simulink model "CAN_Tx"  (R2019b)
settings: Solver=FixedStepDiscrete  StartTime=0.0  StopTime=Inf  RelTol=1e-3  EnableMultiTasking=on
libraries: c2837xDlib x2, drivingvehiclecontroller x1, canmsglib x1, c280xlib x1
settings Model: ExtModeTrigDuration=8  Creator=The MathWorks, Inc.  LastModifiedBy=hang
settings DataIOCC: LimitDataPoints=on  SaveFormat=Array  SaveOutput=off  SaveTime=off  ReturnWorkspaceOutputs=off
settings OptimizationCC: DefaultUnderspecifiedDataType=single  ExpressionDepthLimit=2147483647  LifeSpan=1  MaxStackSize=1024  DenormalBehavior=FlushToZero  EfficientTunableParamExpr=on
settings DebuggingCC: UnderspecifiedInitializationDetection=Classic  MergeDetectMultiDrivingBlocksExec=none  SolverPrmCheckMsg=warning  FcnCallInpInsideContextMsg=warning  AllowSymbolicDim=off  StateNameClashWarn=warning  SFUnexpectedBacktrackingDiag=warning  SFNoUnconditionalDefaultTransitionDiag=warning  SFExecutionAtInitializationDiag=none  ArithmeticOperatorsInVariantConditions=warning
settings HardwareCC: ProdBitPerChar=16  ProdBitPerInt=16  ProdBitPerPointer=32  ProdBitPerSizeT=32  ProdBitPerPtrDiffT=32  ProdLargestAtomicInteger=Integer  ProdLargestAtomicFloat=None  ProdWordSize=16  ProdLongLongMode=on  ProdHWDeviceType=Texas Instruments->C2000
settings ModelReferenceCC: PropagateSignalLabelsOutOfModel=off
settings SFSimCC: SimUseLocalCustomCode=off  MATLABDynamicMemAlloc=off  CustomCodeUndefinedFunction=UseInterfaceOnly
settings RTWCC: SystemTargetFile=ert.tlc  HardwareBoard=TI Delfino F28379D LaunchPad  TemplateMakefile=ert_default_tmf  RTWUseLocalCustomCode=off  Toolchain=Texas Instruments Code Composer Studio (C2000)
settings CodeAppCC: IgnoreCustomStorageClasses=off  CustomSymbolStrType=$N$R$M  StateflowObjectComments=on  InternalIdentifier=Classic
settings ERTTargetCC: CodeReplacementLibrary=TI C28x  MultiwordLength=2048  ExtModeStaticAllocSize=10000  ConvertIfToSwitch=off  SuppressUnreachableDefaultCases=off
settings ConfigComp: CovMetricSettings=dw  CovHtmlReporting=on  CovSaveCumulativeToWorkspaceVar=on  CovSaveSingleToWorkspaceVar=on  CovExternalEMLEnable=off

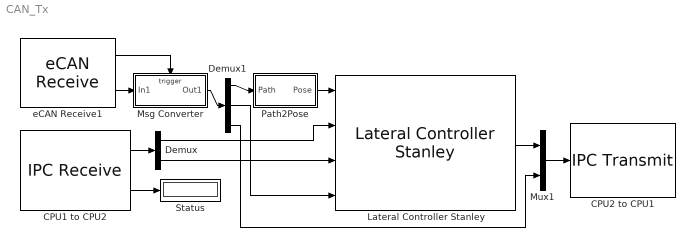
== system CAN_Tx ==
  CPU1 to CPU2 : c2837xDlib/IPC Receive  SelectChannel=1  DataType=uint32  DataLength=1  EnableBlocking=off  SampleTime=0.2
      settings: SourceProductName=Embedded Coder Support Package for Texas Instruments C2000 Processors  SourceProductBaseCode=TIC2000
  CPU2 to CPU1 : c2837xDlib/IPC Transmit  SelectChannel=0  EnableBlocking=off
      settings: SourceProductName=Embedded Coder Support Package for Texas Instruments C2000 Processors  SourceProductBaseCode=TIC2000
  Demux : Demux  Outputs=2
  Demux1 : Demux  Outputs=3
  Lateral Controller Stanley : drivingvehiclecontroller/Lateral Controller Stanley  ModelType=Kinematic bicycle model  PositionGainF=2.5  PositionGainR=2.5  YawRateGain=0.2  DelayGain=0.2  VehicleMass=1575  Lf=1.2  Lr=1.6  TireStiffness=19000  Wheelbase=2.8  MaxSteeringAngle=35
      settings: SourceProductName=Automated Driving Toolbox  SourceProductBaseCode=DR
  Msg Converter : Subsystem  TreatAsAtomicUnit=on
  Mux1 : Mux  Inputs=2
  Path2Pose : Subsystem
  Status : Display
  eCAN Receive1 : c280xlib/eCAN Receive  chipFamily=C280x  useModule=eCAN_B  mailboxNo=0  messageID=bin2dec('1')  messageType=Standard (11-bit identifier)  sampleTime=0.005  dataType=CAN_MESSAGE_TYPE  initValue=0  outputMessageLength=off  outputMessageTimeStamp=off  postInterrupt=off  interruptLine=0
      settings: SourceProductName=Embedded Coder Support Package for Texas Instruments C2000 Processors  SourceProductBaseCode=TIC2000
  wires:
  eCAN Receive1/2 -> Msg Converter/1(In1)
  eCAN Receive1/1 -> Msg Converter/Trigger
  Path2Pose/1(Pose) -> Lateral Controller Stanley/1
  CPU1 to CPU2/1 -> Demux/1
  Demux/1 -> Lateral Controller Stanley/2
  Demux/2 -> Lateral Controller Stanley/3
  CPU1 to CPU2/2 -> Status/1
  Mux1/1 -> CPU2 to CPU1/1
  Lateral Controller Stanley/1 -> Mux1/1
  Demux1/1 -> Path2Pose/1(Path)
  Msg Converter/1(Out1) -> Demux1/1
  Demux1/2 -> Lateral Controller Stanley/4
  Demux1/3 -> Mux1/2

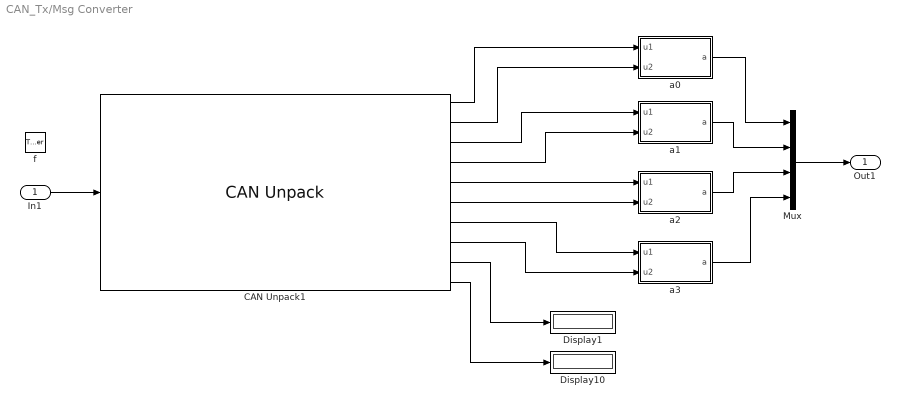
== system CAN_Tx/Msg Converter ==
  In1 : Inport
  f : TriggerPort  TriggerType=function-call  VariantControl=Variant
  CAN Unpack1 : canmsglib/CAN Unpack  MsgList=(none)  MsgName=CAN Msg  MsgIDType=Standard (11-bit identifier)  MsgIdentifier=bin2dec('1')  MsgLength=8  SignalInfo={ 'Signal1', '0', '8', 'LE', 'unsigned', 'Standard', '0', '1', '0', '0', '255'; 'Signal2', '8', '8', 'LE', 'unsigned', 'Standard', '0', '1', '0', '0', '255'; 'Signal3', '16', '8', 'LE', 'unsigned', 'Standard', '0', '1', '0', '0', '255'; 'Signal4', '24', '8', 'LE', 'unsigned', 'Standard', '0', '1', '0', '0', '255'; 'Signal5', '32', '8', 'LE', 'unsigned', 'Standard', '0', '1', '0', '0', '255'; 'Signal6', '40', '8', 'LE', 'unsigned', 'Standard', '0', '1', '0', '0', '255'; 'Signal7', '48', '8', 'LE', 'unsigned', 'Standard', '0', '1', '0', '0', '255'; 'Signal8', '56', '8', 'LE', 'unsigned', 'Standard', '0', '1', '0', '0', '255' }  IDPort=off  TimestampPort=off  ErrorPort=off  RemotePort=off  LengthPort=on  StatusPort=on  ApplyMinMax=off
      settings: SourceProductName=Vehicle Network Toolbox  SourceProductBaseCode=VN
  Display1 : Display
  Display10 : Display
  Mux : Mux
  a0 : MATLAB Function  TreatAsAtomicUnit=on
  a1 : MATLAB Function  TreatAsAtomicUnit=on
  a2 : MATLAB Function  TreatAsAtomicUnit=on
  a3 : MATLAB Function  TreatAsAtomicUnit=on
  Out1 : Outport
  wires:
  In1/1 -> CAN Unpack1/1
  CAN Unpack1/9 -> Display1/1
  CAN Unpack1/10 -> Display10/1
  CAN Unpack1/2 -> a0/2(u2)
  CAN Unpack1/1 -> a0/1(u1)
  CAN Unpack1/3 -> a1/1(u1)
  CAN Unpack1/4 -> a1/2(u2)
  CAN Unpack1/5 -> a2/1(u1)
  CAN Unpack1/6 -> a2/2(u2)
  CAN Unpack1/7 -> a3/1(u1)
  CAN Unpack1/8 -> a3/2(u2)
  a0/1(a) -> Mux/1
  a1/1(a) -> Mux/2
  a2/1(a) -> Mux/3
  a3/1(a) -> Mux/4
  Mux/1 -> Out1/1

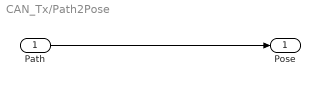
== system CAN_Tx/Path2Pose ==
  Path : Inport
  Pose : Outport
  wires:
  Path/1 -> Pose/1

== matlab function CAN_Tx/Msg Converter/a1 ==
  data: u1 input; a output; u2 input
function a = fcn(u1, u2)

% hex2bin(u1) % high 8-bit
% hex2bin(u2) % low 8-bit

a = uint16(256*u1 + u2);

== matlab function CAN_Tx/Msg Converter/a0 ==
  data: u1 input; a output; u2 input
function a = fcn(u1, u2)

% hex2bin(u1) % high 8-bit
% hex2bin(u2) % low 8-bit

a = uint16(256*u1 + u2);

== matlab function CAN_Tx/Msg Converter/a2 ==
  data: u1 input; a output; u2 input
function a = fcn(u1, u2)

% hex2bin(u1) % high 8-bit
% hex2bin(u2) % low 8-bit

a = uint16(256*u1 + u2);

== matlab function CAN_Tx/Msg Converter/a3 ==
  data: u1 input; a output; u2 input
function a = fcn(u1, u2)

% hex2bin(u1) % high 8-bit
% hex2bin(u2) % low 8-bit

a = uint16(256*u1 + u2);
